simulink model "Game"  (R2023b)
settings: Solver=FixedStepAuto  StartTime=0.0  StopTime=inf  FixedStep=0.001  RelTol=1e-3
libraries: waijung2_host_serial_port_lib x5
settings Model: Creator=warmx  LastModifiedBy=warmx

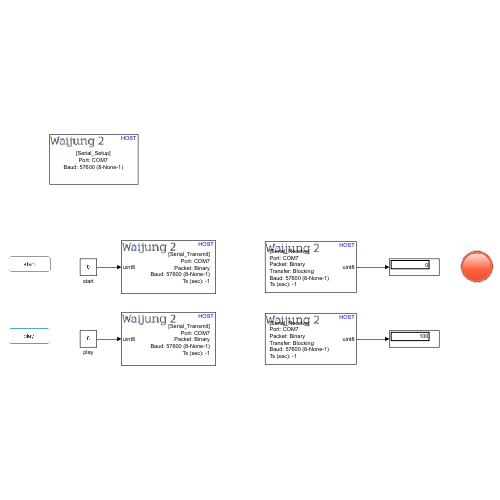
[thumbnail: Simulink's stored preview of the top-level diagram]
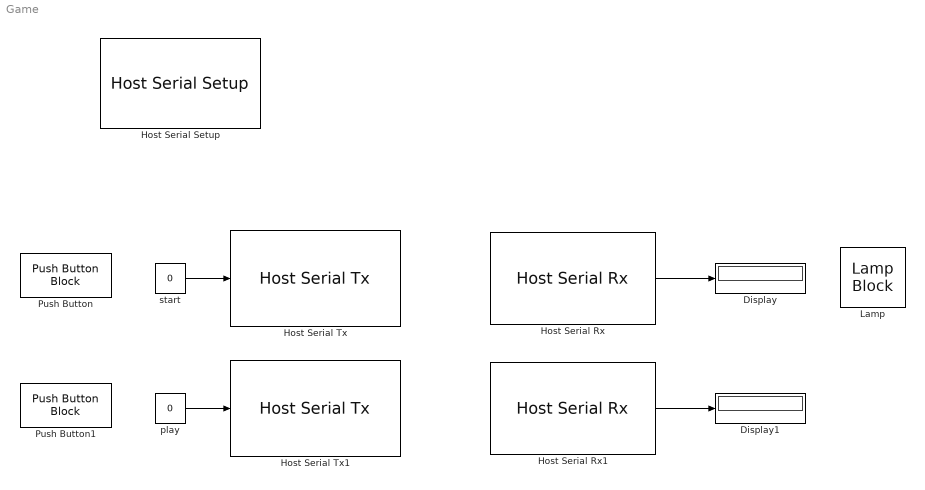
== system Game ==
  Display : Display
  Display1 : Display
  Host Serial Rx : waijung2_host_serial_port_lib/Host Serial Rx  conf=rx  port=<auto>  baudrate=57600  databits=8  parity=None  stopbit=1  flowcontrol=None  transfer=Blocking  timeout=10  packetmode=Binary  enableinitialvalues=off  initialvalues=[]  binheader='61'  binterminator='0A'  porttype_double=0  porttype_single=0  porttype_int8=0  porttype_uint8=1  porttype_int16=0  porttype_uint16=0  porttype_int32=0  porttype_uint32=0  asciiformat='%d,%f'  rx_asciiterminator="CRLF (0x0D 0x0A - \"\\r\\n\")"  tx_asciiterminator="CRLF (0x0D 0x0A - \"\\r\\n\")"  sampletime=-1  enablecustomportlabel=off  cinputportlabel=0  coutputportlabel=A  portpinstr=0  blockid=HostSerialRx  inputporttype=[]  inputportwidth=[]  inputportlabel={}  outputporttype=[3]  outputportwidth=[1]  outputportlabel={'uint8'}  compat=0  optionstring=[]  autoport='COM7'
      settings: SourceProductName=Waijung 2 Blockset
  Host Serial Rx1 : waijung2_host_serial_port_lib/Host Serial Rx  conf=rx  port=<auto>  baudrate=57600  databits=8  parity=None  stopbit=1  flowcontrol=None  transfer=Blocking  timeout=10  packetmode=Binary  enableinitialvalues=off  initialvalues=[]  binheader='62'  binterminator='0A'  porttype_double=0  porttype_single=0  porttype_int8=0  porttype_uint8=1  porttype_int16=0  porttype_uint16=0  porttype_int32=0  porttype_uint32=0  asciiformat='%d,%f'  rx_asciiterminator="CRLF (0x0D 0x0A - \"\\r\\n\")"  tx_asciiterminator="CRLF (0x0D 0x0A - \"\\r\\n\")"  sampletime=-1  enablecustomportlabel=off  cinputportlabel=0  coutputportlabel=A  portpinstr=0  blockid=HostSerialRx1  inputporttype=[]  inputportwidth=[]  inputportlabel={}  outputporttype=[3]  outputportwidth=[1]  outputportlabel={'uint8'}  compat=0  optionstring=[]  autoport='COM7'
      settings: SourceProductName=Waijung 2 Blockset
  Host Serial Setup : waijung2_host_serial_port_lib/Host Serial Setup  conf=setup  port=<auto>  baudrate=57600  databits=8  parity=None  stopbit=1  flowcontrol=None  transfer=Blocking  timeout=2  packetmode=Binary  initialvalues=[]  binheader='7E 7E'  binterminator='03 03'  porttype_double=0  porttype_single=1  porttype_int8=0  porttype_uint8=0  porttype_int16=0  porttype_uint16=0  porttype_int32=0  porttype_uint32=2  asciiformat='%d %u %x'  rx_asciiterminator="CRLF (0x0D 0x0A - \"\\r\\n\")"  tx_asciiterminator="CRLF (0x0D 0x0A - \"\\r\\n\")"  sampletime=-1  enablecustomportlabel=off  cinputportlabel=0  coutputportlabel=A  portpinstr=0  blockid=HostSerialSetup  inputporttype=[]  inputportwidth=[]  inputportlabel={}  outputporttype=[]  outputportwidth=[]  outputportlabel={}  compat=0  optionstring=[]  autoport='COM7'
      settings: SourceProductName=Waijung 2 Blockset
  Host Serial Tx : waijung2_host_serial_port_lib/Host Serial Tx  conf=tx  port=<auto>  baudrate=57600  databits=8  parity=None  stopbit=1  flowcontrol=None  transfer=Blocking  timeout=2  packetmode=Binary  initialvalues=[]  binheader='61'  binterminator='0A'  porttype_double=0  porttype_single=0  porttype_int8=0  porttype_uint8=1  porttype_int16=0  porttype_uint16=0  porttype_int32=0  porttype_uint32=0  asciiformat='%d,%f'  rx_asciiterminator="CRLF (0x0D 0x0A - \"\\r\\n\")"  tx_asciiterminator="CRLF (0x0D 0x0A - \"\\r\\n\")"  sampletime=-1  enablecustomportlabel=off  cinputportlabel=0  coutputportlabel=A  portpinstr=0  blockid=HostSerialTx  inputporttype=[3]  inputportwidth=[1]  inputportlabel={'uint8'}  outputporttype=[]  outputportwidth=[]  outputportlabel={}  compat=0  optionstring=[]  autoport='COM7'
      settings: SourceProductName=Waijung 2 Blockset
  Host Serial Tx1 : waijung2_host_serial_port_lib/Host Serial Tx  conf=tx  port=<auto>  baudrate=57600  databits=8  parity=None  stopbit=1  flowcontrol=None  transfer=Blocking  timeout=2  packetmode=Binary  initialvalues=[]  binheader='62'  binterminator='0A'  porttype_double=0  porttype_single=0  porttype_int8=0  porttype_uint8=1  porttype_int16=0  porttype_uint16=0  porttype_int32=0  porttype_uint32=0  asciiformat='%d,%f'  rx_asciiterminator="CRLF (0x0D 0x0A - \"\\r\\n\")"  tx_asciiterminator="CRLF (0x0D 0x0A - \"\\r\\n\")"  sampletime=-1  enablecustomportlabel=off  cinputportlabel=0  coutputportlabel=A  portpinstr=0  blockid=HostSerialTx1  inputporttype=[3]  inputportwidth=[1]  inputportlabel={'uint8'}  outputporttype=[]  outputportwidth=[]  outputportlabel={}  compat=0  optionstring=[]  autoport='COM7'
      settings: SourceProductName=Waijung 2 Blockset
  Lamp : LampBlock  LabelPosition=Hide
  Push Button : PushButtonBlock  ButtonText=start  OffValue=0.000000
  Push Button1 : PushButtonBlock  ButtonText=play  OffValue=0.000000
  play : Constant  Value=0  OutDataTypeStr=uint8
  start : Constant  Value=0  OutDataTypeStr=uint8
  wires:
  start/1 -> Host Serial Tx/1
  play/1 -> Host Serial Tx1/1
  Host Serial Rx/1 -> Display/1
  Host Serial Rx1/1 -> Display1/1
